simulink model "c28069pmsmfoc_cla"  (R2021b)
settings: Solver=FixedStepDiscrete  StartTime=0.0  StopTime=inf  RelTol=1e-3  EnableMultiTasking=on
PreLoadFcn:
  | c28069pmsmfoc_data;
model workspace (MAT data in the model file):
  encoderResolution = 2000
  hallOffset = '0.5'
  indexOffset = 850
  polePairs = '4'
values from neighbouring files (symbols this model uses):
  Hall_position_offset = 0.57    [c28027pmsmfoc_data.m]    (also in c28035pmsmfoc_data.m; c28035pmsmfoc_data_cla.m; c28069pmsmfoc_data.m)
  PWM_Counter_Period = CPU_frequency/PWM_frequency/2    (= 1500)    [c28027pmsmfoc_data.m]    (also in c28035pmsmfoc_data.m; c28035pmsmfoc_data_cla.m = 2500; c28069pmsmfoc_data.m = 2250)
  Speed_per_unit_scaler = 1200    [c28027pmsmfoc_data.m]    (also in c28035pmsmfoc_data.m; c28035pmsmfoc_data_cla.m = 600; c28069pmsmfoc_data.m)
  Speed_rpm_scaler = 60*CPU_frequency/Pole_pairs/2    (= 450000000)    [c28027pmsmfoc_data.m]    (also in c28035pmsmfoc_data.m; c28035pmsmfoc_data_cla.m; c28069pmsmfoc_data.m = 675000000)
undefined symbols (not defined in the file or in its folder): codertarget, Down, GPTRIP1SEL, GPTRIP2SEL, TZ1, TZ2, Up
libraries: idelinklib_common x12, c2802xlib x7, tiiqmathlib x7, hall_sensor_lib x7, c280xlib x3, c2803xlib x2, simulink x2, etargetslib x2, demo_controls x1, c2806xlib x1, c2000lib x1
(part 2 of 3)

== system c28069pmsmfoc_cla/FOC Algorithm/Torque Control Algorithm/Atomic Hall Reading ==
  Disable Interrupts for Atomic Read : Subsystem  mask(System Outputs){ShowInLibBrowser=0}
      mask prompts: ShowInLibBrowser "Simulink:masks:CustCodeMaskParam1_MP"
      settings: CopyFcn=cccopyfcn(gcb)  OpenFcn=ccopenfcn('System Outputs Function')
      mask Help: eval('feval(''rtwprivate'',''rtwhelpview'',''rtw_sys_outputs_block'')');
      mask Display: disp('System\nOutputs');
  Read Global Direction Flag : DataStoreRead  DataStoreName=Global_direction  IndexOptions=Index vector (dialog)  Indices=1  OutputSizes=1
  Read Global Speed : DataStoreRead  DataStoreName=Global_speed  IndexOptions=Index vector (dialog)  Indices=1  OutputSizes=1
  Read Global Speed and Direction Valid Flag : DataStoreRead  DataStoreName=Global_speed_and_direction_valid_flag  IndexOptions=Index vector (dialog)  Indices=1  OutputSizes=1
  Read Hall Watchdog : DataStoreRead  DataStoreName=Hall_Watchdog  IndexOptions=Index vector (dialog)  Indices=1  OutputSizes=1
  Read Halls : hall_sensor_lib/Read_halls  sample_time=-1
      settings: SourceProductBaseCode=TIC2000
  Update Hall Watchdog : Subsystem
  Direction : Outport
  Valid Flag : Outport  Port=2
  Speed : Outport  Port=3
  Halls : Outport  Port=4
  Hall Watchdog : Outport  Port=5
  wires:
  Read Hall Watchdog/1 -> Hall Watchdog/1, Update Hall Watchdog/1(In1)
  Read Halls/1 -> Halls/1
  Read Global Speed/1 -> Speed/1
  Read Global Speed and Direction Valid Flag/1 -> Valid Flag/1
  Read Global Direction Flag/1 -> Direction/1

== system c28069pmsmfoc_cla/FOC Algorithm/Torque Control Algorithm/Direction Scaling ==
  Dir : Inport
  Bias : Bias  Bias=1
  Binary Direction : Outport
  wires:
  Bias/1 -> Binary Direction/1
  Dir/1 -> Bias/1

== system c28069pmsmfoc_cla/FOC Algorithm/Torque Control Algorithm/Generating Space Vectors ==
  Speed/Pos/Dir : Inport
  Ia : Inport  Port=2
  Ib : Inport  Port=3
  Iq Desired : Inport  Port=4
  CLA Task : c2806xlib/CLA Task  taskNumber=1  intSource=Software  sampleTime=-1  claType=0  softTrigSelected=1  enableInterrupt=on
      settings: SourceProductBaseCode=TIC2000
  Data Type Conversion{1..3,7} (4 alike) : DataTypeConversion  OutDataTypeStr=single
  Generating Raw Space Vectors : Subsystem  Tag=ClaSubsystem  InitFcn=codertarget.registry.registerC28xNonPeripheralBlocks(gcb)  TreatAsAtomicUnit=on  RTWFileName=sample_cla  mask(c28x CLA Subsystem){}
      settings: CopyFcn=codertarget.registry.setC28xCLASubSystem(gcb)  OpenFcn=open_system(gcbh,'force')  RTWSystemCode=Nonreusable function  RTWFileNameOpts=User specified  FunctionWithSeparateData=on  RTWMemSecFuncInitTerm=C28xFunction  RTWMemSecFuncExecute=ClaFunction  RTWMemSecDataConstants=Cla1DataRam  RTWMemSecDataInternal=Cla1DataRam  RTWMemSecDataParameters=Cla1DataRam
      mask Display: color('black'); text(0.50, 0.12, 'CLA Subsystem', 'horizontalAlignment','center');
  Selector : Selector  InputPortWidth=3  IndexOptions=Index vector (dialog)  Indices=2  OutputSizes=1
  wires:
  Ib/1 -> Data Type Conversion1/1
  Data Type Conversion2/1 -> Generating Raw Space Vectors/1(Ia)
  Iq Desired/1 -> Data Type Conversion7/1
  CLA Task/1 -> Generating Raw Space Vectors/Trigger
  Data Type Conversion1/1 -> Generating Raw Space Vectors/2(Ib)
  Data Type Conversion3/1 -> Generating Raw Space Vectors/3(position)
  Data Type Conversion7/1 -> Generating Raw Space Vectors/4(iQ_desired)
  Selector/1 -> Data Type Conversion3/1
  Ia/1 -> Data Type Conversion2/1
  Speed/Pos/Dir/1 -> Selector/1

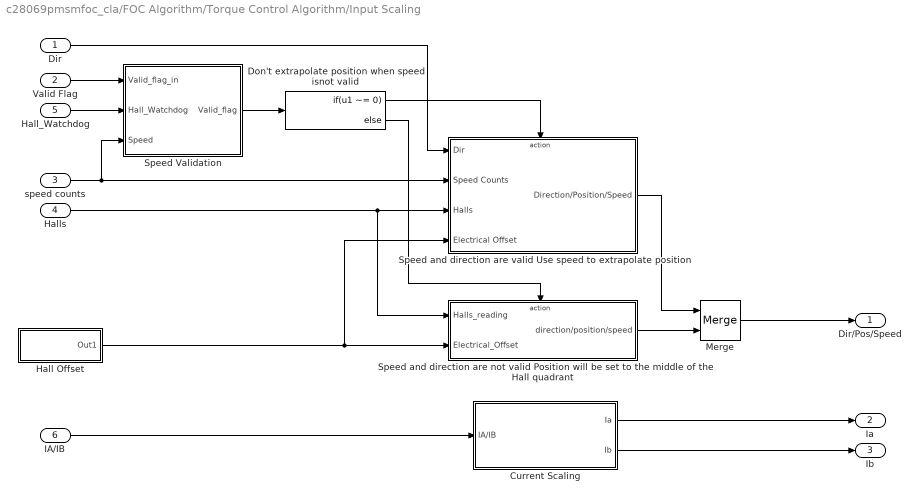
== system c28069pmsmfoc_cla/FOC Algorithm/Torque Control Algorithm/Input Scaling ==
  Dir : Inport
  Valid Flag : Inport  Port=2
  speed counts : Inport  Port=3
  Halls : Inport  Port=4
  Hall_Watchdog : Inport  Port=5
  IA/IB : Inport  Port=6
  Current Scaling : Subsystem
  Don't extrapolate position when speed isnot valid : If  IfExpression=u1 ~= 0
  Hall Offset : Subsystem
  Merge : Merge
  Speed Validation : Subsystem
  Speed and direction are not valid Position will be set to the middle of the Hall quadrant : Subsystem  TreatAsAtomicUnit=on
  Speed and direction are valid Use speed to extrapolate position : Subsystem  TreatAsAtomicUnit=on
  Dir/Pos/Speed : Outport  InitialOutput=0
  Ia : Outport  Port=2
  Ib : Outport  Port=3
  wires:
  IA/IB/1 -> Current Scaling/1(IA/IB)
  Current Scaling/2(Ib) -> Ib/1
  Current Scaling/1(Ia) -> Ia/1
  Hall_Watchdog/1 -> Speed Validation/2(Hall_Watchdog)
  Speed and direction are not valid Position will be set to the middle of the Hall quadrant/1(direction/position/speed) -> Merge/2
  Speed and direction are valid Use speed to extrapolate position/1(Direction/Position/Speed) -> Merge/1
  Speed Validation/1(Valid_flag) -> Don't extrapolate position when speed isnot valid/1
  Merge/1 -> Dir/Pos/Speed/1
  Don't extrapolate position when speed isnot valid/1 -> Speed and direction are valid Use speed to extrapolate position/Action
  Valid Flag/1 -> Speed Validation/1(Valid_flag_in)
  Halls/1 -> Speed and direction are valid Use speed to extrapolate position/3(Halls), Speed and direction are not valid Position will be set to the middle of the Hall quadrant/1(Halls_reading)
  speed counts/1 -> Speed Validation/3(Speed), Speed and direction are valid Use speed to extrapolate position/2(Speed Counts)
  Dir/1 -> Speed and direction are valid Use speed to extrapolate position/1(Dir)
  Hall Offset/1(Out1) -> Speed and direction are not valid Position will be set to the middle of the Hall quadrant/2(Electrical_Offset), Speed and direction are valid Use speed to extrapolate position/4(Electrical Offset)
  Don't extrapolate position when speed isnot valid/2 -> Speed and direction are not valid Position will be set to the middle of the Hall quadrant/Action

== system c28069pmsmfoc_cla/FOC Algorithm/Torque Control Algorithm/Send to DAC 3 ==
  Position : Inport
  Bitwise Operator : simulink/Logic and Bit Operations/Bitwise Operator  logicop=AND  UseBitMask=on  BitMask=hex2dec('0FFF')  BitMaskRealWorld=Stored Integer
  DAC 3 : c2802xlib/ePWM  PwmType=C2000  useModule=ePWM5  ePWMxLINKTBPRD=Not Linked  periodUnits=Clock cycles  timerSource=Specify via dialog  timerPeriod_clk=4095  timerPeriod_sec=64000  tbshadow=Counter equals to zero  countingMode=Up  phaseActiveEnable=Disable  phaseDirection=Count down after sync  phaseActive=0  synchronizationEnable=off  dcaevt1Sync=off  dcbevt1Sync=off  synchronizationOption=Disable  perSynchronizationOption=Counter equals to period (CTR=PRD)  clockPrescale=1  HSclockPrescale=1  enswap=off  ePWMxAStatus=on  ePWMxAactionLogic1=Do nothing  ePWMxAactionLogic2=Set  ePWMxAactionLogic3=Clear  ePWMxAactionLogic4=Do nothing  ePWMxAactionLogic5=Do nothing  ePWMxAactionLogic6=Do nothing  ePWMxACSFenable=off  ePWMxACSFvalue=Forcing disable  ePWMxASFreload=Zero  ePWMxBStatus=off  ePWMxBactionLogic1=Do nothing  ePWMxBactionLogic2=Set  ePWMxBactionLogic3=Do nothing  ePWMxBactionLogic4=Do nothing  ePWMxBactionLogic5=Clear  ePWMxBactionLogic6=Do nothing  ePWMxBCSFenable=off  ePWMxBCSFvalue=Forcing disable  ePWMxBSFreload=Zero  ePWNxBOutWay=off  ePWMxLINKCMPA=Not Linked  CMPAUnits=Clock cycles  CMPASource=Input port  CMPAValue_per=32000  CMPAValue_clk=0  enCMPAshadow=Counter equals to zero (CTR=Zero)  ePWMxLINKCMPB=Not Linked  CMPBUnits=Clock cycles  CMPBSource=Specify via dialog  CMPBValue_per=50  CMPBValue_clk=0  enCMPBshadow=Counter equals to zero (CTR=Zero)  ePWMxLINKCMPC=Not Linked  CMPCUnits=Clock cycles  CMPCSource=Specify via dialog  CMPCValue_per=50  CMPCValue_clk=32000  enCMPCshadow=Counter equals to zero (CTR=Zero)  ePWMxLINKCMPD=Not Linked  CMPDUnits=Clock cycles  CMPDSource=Specify via dialog  CMPDValue_per=50  CMPDValue_clk=32000  enCMPDshadow=Counter equals to zero (CTR=Zero)  enableDBePWMxA=off  enableDBePWMxB=off  enhalfcycle=off  DBpolarity=Active high (AH)  DBedgeDelay=Positive  DBSource_ePWMxA=ePWMxA  DBSource_ePWMxB=ePWMxA  DBPeriodUnits=Clock cycles  DBperiodSource=Specify via dialog  REDperiod=0  FEDperiod=0  REDperiod_sec=0  FEDperiod_sec=0  LoadModeDBRED=Immediate without using shadow  LoadModeDBFED=Immediate without using shadow  adcstartModuleA=off  adcrequestEventA=First event  adcstartEventA=Digital Compare Module A Event 1 start of conversion (DCAEVT1.soc)  adcstartEventA_type2=Digital Compare Module A Event 1 start of conversion (DCAEVT1.soc)  adcstartModuleB=off  adcrequestEventB=First event  adcstartEventB=Counter equals to zero (CTR=Zero)  adcstartEventB_type2=Counter equals to zero (CTR=Zero)  intEn=off  intPrd=First event  intSel=Counter equals to zero (CTR=Zero)  intSel_type2=Counter equals to zero (CTR=Zero)  hrpe=off  enHRPWM=off  HRPWM_LoadMode=Counter equals to period (CTR=PRD)  HRPWM_CTLMode=Duty or Period control mode  HRPWM_EDGMode=Both edge  hrpeb=off  enHRPWMB=off  HRPWM_LoadModeB=Counter equals to zero (CTR=ZERO)  HRPWM_CTLModeB=Duty or Period control mode  HRPWM_EDGModeB=Both edge  enHRDBRED=off  enHRDBFED=off  enSFO=on  enautoconv=on  chopperEnable=off  chopperFrequency=1  chopperFirstwidth=1  chopperDuty=12.5%  tripZonesource=Specify via dialog  tzselOSHT1=off  tzselOSHT2=off  tzselOSHT3=off  tzselOSHDCAEV1=off  tzselOSHDCBEV1=off  tzselCBC1=off  tzselCBC2=off  tzselCBC3=off  tzselCBCDCAEV2=off  tzselCBCDCBEV2=off  tzselOSHT4=off  tzselOSHT5=off  tzselOSHT6=off  tzselCBC4=off  tzselCBC5=off  tzselCBC6=off  enTzOstIntr=off  enTzCbcIntr=off  enTzDCAEVT1Intr=off  enTzDCAEVT2Intr=off  enTzDCBEVT1Intr=off  enTzDCBEVT2Intr=off  ePWMxAforced=No action  ePWMxBforced=No action  DCAEVT1forced=No action  DCBEVT1forced=No action  DCAEVT2forced=No action  DCBEVT2forced=No action  dcah=Trip Zone 1 input (TZ1)  dcal=Trip Zone 2 input (TZ2)  dcbh=Trip Zone 1 input (TZ1)  dcbl=Trip Zone 2 input (TZ2)  dcah_type2=GPTRIP1SEL/(TZ1)  dcal_type2=GPTRIP2SEL/(TZ2)  dcbh_type2=GPTRIP1SEL/(TZ1)  dcbl_type2=GPTRIP2SEL/(TZ2)  gendcaevt1=Event disabled  gendcaevt2=Event disabled  gendcbevt1=Event disabled  gendcbevt2=Event disabled  dcaevt1src=DCAEVT1 with sync  dcaevt2src=DCAEVT2 with sync  dcbevt1src=DCBEVT1 with sync  dcbevt2src=DCBEVT2 with sync  pulsesel=Counter equals to zero (CTR=Zero)  blankinv=off  blankoffset=0  blankwidth=0  evsrcsel=Filtered version of DCAEVT1 (DCAEVT1FILT)  encape=off
  Data Type Conversion : DataTypeConversion  OutDataTypeStr=uint16  ConvertRealWorld=Stored Integer (SI)
  Shift Arithmetic2 : ArithShift  BitShiftNumber=5  BitShiftDirection=Right
  wires:
  Shift Arithmetic2/1 -> Data Type Conversion/1
  Data Type Conversion/1 -> Bitwise Operator/1
  Position/1 -> Shift Arithmetic2/1
  Bitwise Operator/1 -> DAC 3/1

== system c28069pmsmfoc_cla/FOC Algorithm/Torque Control Algorithm/Speed IIR filter ==
  Speed : Inport
  Add : Sum  Inputs=+-
  Add1 : Sum
  Constant1 : Constant  OutDataTypeStr=fixdt(1,32,17)
  Constant2 : Constant  Value=.01  OutDataTypeStr=fixdt(1,32,17)
  Product : Product  OutDataTypeStr=Inherit: Same as first input
  Product1 : Product  OutDataTypeStr=Inherit: Same as first input
  Unit Delay : UnitDelay  SampleTime=-1  HasFrameUpgradeWarning=on
  Filtered speed : Outport
  wires:
  Speed/1 -> Product/1
  Add1/1 -> Unit Delay/1, Filtered speed/1
  Constant1/1 -> Add/1
  Constant2/1 -> Product/2, Add/2
  Product/1 -> Add1/1
  Add/1 -> Product1/1
  Unit Delay/1 -> Product1/2
  Product1/1 -> Add1/2

== system c28069pmsmfoc_cla/Hall Sensor A/Overflow Detection/No overflow detected ==
  old_validate : Inport
  Action Port : ActionPort  ActionPortLabel=else
  Unit Delay3 : UnitDelay  SampleTime=-1  HasFrameUpgradeWarning=on
  New_valid_flag : Outport
  wires:
  old_validate/1 -> Unit Delay3/1
  Unit Delay3/1 -> New_valid_flag/1

== system c28069pmsmfoc_cla/Hall Sensor A/Overflow Detection/Overflow detected ==
  Action Port : ActionPort  ActionPortLabel=if(u1 ~= 0)
  Constant : Constant  Value=0  OutDataTypeStr=uint16
  Constant2 : Constant  Value=0  OutDataTypeStr=uint16
  Data Store : DataStoreWrite  DataStoreName=Global_speed_and_direction_valid_flag  IndexOptions=Index vector (dialog)  Indices=1  OutputSizes=1
  New_valid_flag : Outport
  wires:
  Constant/1 -> New_valid_flag/1
  Constant2/1 -> Data Store/1

== system c28069pmsmfoc_cla/Hall Sensor A/Update Speed and Direction/update_speed ==
  In1 : Inport
  Action Port : ActionPort  ActionPortLabel=if(u1 ~= 0)
  Data Store Write3 : DataStoreWrite  DataStoreName=Global_speed  IndexOptions=Index vector (dialog)  Indices=1  OutputSizes=1
  wires:
  In1/1 -> Data Store Write3/1

== system c28069pmsmfoc_cla/Hall Sensor B/Overflow Detection/No overflow detected ==
  old_validate : Inport
  Action Port : ActionPort  ActionPortLabel=else
  Unit Delay3 : UnitDelay  SampleTime=-1  HasFrameUpgradeWarning=on
  New_valid_flag : Outport
  wires:
  Unit Delay3/1 -> New_valid_flag/1
  old_validate/1 -> Unit Delay3/1

== system c28069pmsmfoc_cla/Hall Sensor B/Overflow Detection/Overflow detected ==
  Action Port : ActionPort  ActionPortLabel=if(u1 ~= 0)
  Constant : Constant  Value=0  OutDataTypeStr=uint16
  Constant2 : Constant  Value=0  OutDataTypeStr=uint16
  Data Store : DataStoreWrite  DataStoreName=Global_speed_and_direction_valid_flag  IndexOptions=Index vector (dialog)  Indices=1  OutputSizes=1
  New_valid_flag : Outport
  wires:
  Constant2/1 -> Data Store/1
  Constant/1 -> New_valid_flag/1

== system c28069pmsmfoc_cla/Hall Sensor B/Update Speed and Direction/update_speed ==
  In1 : Inport
  Action Port : ActionPort  ActionPortLabel=if(u1 ~= 0)
  Data Store Write3 : DataStoreWrite  DataStoreName=Global_speed  IndexOptions=Index vector (dialog)  Indices=1  OutputSizes=1
  wires:
  In1/1 -> Data Store Write3/1

== system c28069pmsmfoc_cla/Hall Sensor C/Overflow Detection/No overflow detected ==
  old_validate : Inport
  Action Port : ActionPort  ActionPortLabel=else
  Unit Delay3 : UnitDelay  SampleTime=-1  HasFrameUpgradeWarning=on
  New_valid_flag : Outport
  wires:
  old_validate/1 -> Unit Delay3/1
  Unit Delay3/1 -> New_valid_flag/1

== system c28069pmsmfoc_cla/Hall Sensor C/Overflow Detection/Overflow detected ==
  Action Port : ActionPort  ActionPortLabel=if(u1 ~= 0)
  Constant : Constant  Value=0  OutDataTypeStr=uint16
  Constant2 : Constant  Value=0  OutDataTypeStr=uint16
  Data Store : DataStoreWrite  DataStoreName=Global_speed_and_direction_valid_flag  IndexOptions=Index vector (dialog)  Indices=1  OutputSizes=1
  New_valid_flag : Outport
  wires:
  Constant/1 -> New_valid_flag/1
  Constant2/1 -> Data Store/1

== system c28069pmsmfoc_cla/Hall Sensor C/Update Speed and Direction/update_speed ==
  In1 : Inport
  Action Port : ActionPort  ActionPortLabel=if(u1 ~= 0)
  Data Store Write3 : DataStoreWrite  DataStoreName=Global_speed  IndexOptions=Index vector (dialog)  Indices=1  OutputSizes=1
  wires:
  In1/1 -> Data Store Write3/1

== system c28069pmsmfoc_cla/Speed Controller/PID Controller/UD_REG3 ==
  up_reg3 : Inport
  PrevOut : Inport  Port=2
  Constant : Constant  Value=derivativeGain  OutDataTypeStr=Inherit: Inherit via back propagation
  Product : Product  OutDataTypeStr=Inherit: Same as first input
  Sum2 : Sum  Inputs=+-
  Out1 : Outport
  wires:
  Constant/1 -> Product/1
  Product/1 -> Out1/1
  Sum2/1 -> Product/2
  PrevOut/1 -> Sum2/2
  up_reg3/1 -> Sum2/1

== system c28069pmsmfoc_cla/Speed Controller/PID Controller/UI_REG3 ==
  OLD_UI_REG3 : Inport
  up_reg3 : Inport  Port=2
  saterr_reg3 : Inport  Port=3
  Constant : Constant  Value=integralGain  OutDataTypeStr=Inherit: Inherit via back propagation
  Constant1 : Constant  Value=correctionGain  OutDataTypeStr=Inherit: Inherit via back propagation
  Product : Product  OutDataTypeStr=Inherit: Same as first input
  Product1 : Product  OutDataTypeStr=Inherit: Same as first input
  Sum1 : Sum  Inputs=+++
  UI_REG1 : Outport
  wires:
  Constant1/1 -> Product1/1
  saterr_reg3/1 -> Product1/2
  Constant/1 -> Product/1
  up_reg3/1 -> Product/2
  Sum1/1 -> UI_REG1/1
  Product1/1 -> Sum1/3
  Product/1 -> Sum1/2
  OLD_UI_REG3/1 -> Sum1/1

== system c28069pmsmfoc_cla/FOC Algorithm/Torque Control Algorithm/Atomic Hall Reading/Disable Interrupts for Atomic Read ==

== system c28069pmsmfoc_cla/FOC Algorithm/Torque Control Algorithm/Atomic Hall Reading/Update Hall Watchdog ==
  In1 : Inport
  Add : Sum  SaturateOnIntegerOverflow=on
      settings: AttributesFormatString=Saturation: %<SaturateOnIntegerOverflow>
  Constant2 : Constant  OutDataTypeStr=uint16
  Write Hall Watchdog : DataStoreWrite  DataStoreName=Hall_Watchdog  IndexOptions=Index vector (dialog)  Indices=1  OutputSizes=1
  wires:
  Add/1 -> Write Hall Watchdog/1
  Constant2/1 -> Add/2
  In1/1 -> Add/1

== system c28069pmsmfoc_cla/FOC Algorithm/Torque Control Algorithm/Generating Space Vectors/Generating Raw Space Vectors ==
  Ia : Inport
  Ib : Inport  Port=2
  position : Inport  Port=3
  iQ_desired : Inport  Port=4
  function : TriggerPort  TriggerType=function-call  VariantControl=Variant
  Clarke Transformation : Subsystem  InitFcn=tic2000lib_licenseCheck  mask(Clarke Transformation){}
      mask help: This block performs transformation of three-phase quantities into balanced two-phase quadrature quantities. All inputs and outputs are signed 32-bit fixed-point numbers with Q value between 1 and 29.
      mask Help: eval('linkfoundation.util.openBlockHelp(''c28xdmclibclarketransformation'',''ecoder'')');
      mask Display:
      | port_label('input',1,'As');
      | port_label('input',2,'Bs');
      | port_label('Output',1,'Alpha');
      | port_label('Output',2,'Beta');
      | text(0.5,0.15, 'Clarke', 'horizontalalignment','center');
  Data Store Write : DataStoreWrite  DataStoreName=Ta_out  IndexOptions=Index vector (dialog)  Indices=1  OutputSizes=1
  Data Store Write1 : DataStoreWrite  DataStoreName=Tb_out  IndexOptions=Index vector (dialog)  Indices=1  OutputSizes=1
  Data Store Write2 : DataStoreWrite  DataStoreName=Tc_out  IndexOptions=Index vector (dialog)  Indices=1  OutputSizes=1
  Inverse Park Transformation : Subsystem  InitFcn=tic2000lib_licenseCheck  mask(Inverse Park Transformation){}
      mask help: This block performs vector transformation from orthogonal rotating reference frame into orthogonal stationary frame. All inputs and outputs are signed 32-bit fixed-point numbers with Q value between 1 and 29.
      mask Help: eval('linkfoundation.util.openBlockHelp(''c28xdmclibinverseparktransformation'',''ecoder'')');
      mask Display:
      | port_label('input',1,'Ds');
      | port_label('input',2,'Qs');
      | port_label('input',3,'Angle');
      | port_label('Output',1,'Alpha');
      | port_label('Output',2,'Beta');
      | text(0.5,0.15, 'IPark', 'horizontalalignment','center');
  Park Transformation : Subsystem  InitFcn=tic2000lib_licenseCheck  mask(Park Transformation){}
      mask help: This block performs vector transformation from balanced two-phase orthogonal stationary system into orthogonal rotating frame. All inputs and outputs are signed 32-bit fixed-point numbers with Q value between 1 and 29.
      mask Help: eval('linkfoundation.util.openBlockHelp(''c28xdmclibparktransformation'',''ecoder'')');
      mask Display:
      | port_label('input',1,'Alpha');
      | port_label('input',2,'Beta');
      | port_label('input',3,'Angle');
      | port_label('Output',1,'Ds');
      | port_label('Output',2,'Qs');
      | text(0.5,0.15, 'Park', 'horizontalalignment','center');
  SVGen : Subsystem
  control : Subsystem
  wires:
  control/1(Out1) -> Inverse Park Transformation/1(ID)
  iQ_desired/1 -> control/3(Iq desired)  "iQ_des"
  Ib/1 -> Clarke Transformation/2(Ib)  "Ib_in"
  Ia/1 -> Clarke Transformation/1(Ia)  "Ia_in"
  control/2(Out2) -> Inverse Park Transformation/2(IQ)
  Inverse Park Transformation/1(Out1) -> SVGen/1(Ua)
  Clarke Transformation/2(Out2) -> Park Transformation/2(Iq1)
  Clarke Transformation/1(Out1) -> Park Transformation/1(Id1)
  SVGen/3(Tc) -> Data Store Write2/1
  SVGen/1(Ta) -> Data Store Write/1
  position/1 -> Inverse Park Transformation/3(theta), Park Transformation/3(theta1)  "position"
  Inverse Park Transformation/2(Out2) -> SVGen/2(Ub)
  Park Transformation/2(Out4) -> control/2(Vq)
  SVGen/2(Tb) -> Data Store Write1/1
  Park Transformation/1(Out3) -> control/1(Vd)

== system c28069pmsmfoc_cla/FOC Algorithm/Torque Control Algorithm/Input Scaling/Current Scaling ==
  IA/IB : Inport
  Add : Sum  Inputs=-+
  Constant : Constant  Value=[2048 2048]  OutDataTypeStr=int32
  Data Type Conversion : DataTypeConversion  OutDataTypeStr=int32  ConvertRealWorld=Stored Integer (SI)
  Data Type Conversion1 : DataTypeConversion  OutDataTypeStr=fixdt(1,32,17)  ConvertRealWorld=Stored Integer (SI)
  Demux : Demux  Outputs=2
  Shift Arithmetic : ArithShift  BitShiftNumber=-6
  Ia : Outport
  Ib : Outport  Port=2
  wires:
  IA/IB/1 -> Data Type Conversion/1
  Constant/1 -> Add/1
  Data Type Conversion1/1 -> Demux/1
  Shift Arithmetic/1 -> Data Type Conversion1/1
  Add/1 -> Shift Arithmetic/1
  Data Type Conversion/1 -> Add/2
  Demux/2 -> Ib/1
  Demux/1 -> Ia/1

== system c28069pmsmfoc_cla/FOC Algorithm/Torque Control Algorithm/Input Scaling/Hall Offset ==
  Hall_offset : Constant  Value=Hall_position_offset  OutDataTypeStr=fixdt(1,32,17)
  Out1 : Outport
  wires:
  Hall_offset/1 -> Out1/1

== system c28069pmsmfoc_cla/FOC Algorithm/Torque Control Algorithm/Input Scaling/Speed Validation ==
  Valid_flag_in : Inport
  Hall_Watchdog : Inport  Port=2
  Speed : Inport  Port=3
  Constant : Constant  Value=0  OutDataTypeStr=uint16
  Don't trust speed if Hall Watchdog counter is too high. Hall Watchdog is reset at every Hall edge. : Switch  Threshold=65000
  Don't trust speed if it is below 10rpm : Switch  Threshold=Speed_rpm_scaler/10
  Valid_flag : Outport
  wires:
  Don't trust speed if it is below 10rpm/1 -> Don't trust speed if Hall Watchdog counter is too high. Hall Watchdog is reset at every Hall edge./3
  Valid_flag_in/1 -> Don't trust speed if it is below 10rpm/3
  Speed/1 -> Don't trust speed if it is below 10rpm/2
  Don't trust speed if Hall Watchdog counter is too high. Hall Watchdog is reset at every Hall edge./1 -> Valid_flag/1
  Constant/1 -> Don't trust speed if it is below 10rpm/1, Don't trust speed if Hall Watchdog counter is too high. Hall Watchdog is reset at every Hall edge./1
  Hall_Watchdog/1 -> Don't trust speed if Hall Watchdog counter is too high. Hall Watchdog is reset at every Hall edge./2

== system c28069pmsmfoc_cla/FOC Algorithm/Torque Control Algorithm/Input Scaling/Speed and direction are not valid Position will be set to the middle of the Hall quadrant ==
  Halls_reading : Inport
  Electrical_Offset : Inport  Port=2
  Action Port : ActionPort  ActionPortLabel=else
  Add : Sum
  Direction : Constant  Value=0  OutDataTypeStr=fixdt(1,32,17)
  Extract position from Halls reading. No speed extrapolaiton : Subsystem
  Mux1 : Mux  Inputs=3
  Speed : Constant  Value=0  OutDataTypeStr=fixdt(1,32,17)
  direction/position/speed : Outport  InitialOutput=0
  wires:
  Speed/1 -> Mux1/3
  Electrical_Offset/1 -> Add/2
  Add/1 -> Mux1/2
  Extract position from Halls reading. No speed extrapolaiton/1(Raw position) -> Add/1
  Mux1/1 -> direction/position/speed/1
  Direction/1 -> Mux1/1
  Halls_reading/1 -> Extract position from Halls reading. No speed extrapolaiton/1(Halls_reading)

== system c28069pmsmfoc_cla/FOC Algorithm/Torque Control Algorithm/Input Scaling/Speed and direction are valid Use speed to extrapolate position ==
  Dir : Inport
  Speed Counts : Inport  Port=2
  Halls : Inport  Port=3
  Electrical Offset : Inport  Port=4
  Action Port : ActionPort  ActionPortLabel=if(u1 ~= 0)
  Data Type Conversion1 : DataTypeConversion  OutDataTypeStr=fixdt(1,32,17)  ConvertRealWorld=Stored Integer (SI)
  Data Type Conversion2 : DataTypeConversion  OutDataTypeStr=fixdt(1,32,17)
  Demux : Demux  Outputs=2
  Extract Position from Halls : Subsystem
  Extrapolate position : Subsystem
  Mux2 : Mux  Inputs=3
  Per unit speed calcualtion : Subsystem
  Direction/Position/Speed : Outport  InitialOutput=0
  wires:
  Mux2/1 -> Direction/Position/Speed/1
  Data Type Conversion2/1 -> Mux2/1
  Demux/2 -> Extrapolate position/3(offset)
  Demux/1 -> Extrapolate position/2(Counter)
  Extrapolate position/1(Position) -> Mux2/2
  Dir/1 -> Data Type Conversion2/1, Per unit speed calcualtion/1(Dir), Extract Position from Halls/1(Direction)
  Electrical Offset/1 -> Extrapolate position/4(electrical offset)
  Per unit speed calcualtion/1(Per Unit Speed) -> Mux2/3
  Data Type Conversion1/1 -> Extrapolate position/1(Speed Counts), Per unit speed calcualtion/2(Speed counts)
  Halls/1 -> Extract Position from Halls/2(Halls)
  Extract Position from Halls/1(Counter/Offset) -> Demux/1
  Speed Counts/1 -> Data Type Conversion1/1

== system c28069pmsmfoc_cla/FOC Algorithm/Torque Control Algorithm/Generating Space Vectors/Generating Raw Space Vectors/Clarke Transformation ==
  Ia : Inport
  Ib : Inport  Port=2
  1 : Constant  Value=0.57735026918963  OutDataTypeStr=Inherit: Inherit via back propagation
  2 : Constant  Value=2  OutDataTypeStr=Inherit: Inherit via back propagation  SampleTime=Inf
  Product : Product  OutDataTypeStr=single
  Product1 : Product  OutDataTypeStr=Inherit: Same as first input
  Sum1 : Sum  Inputs=|++  OutDataTypeStr=Inherit: Same as first input
  Out1 : Outport
  Out2 : Outport  Port=2
  wires:
  Ib/1 -> Product/2
  Ia/1 -> Out1/1, Sum1/1
  Sum1/1 -> Product1/2
  2/1 -> Product/1
  Product1/1 -> Out2/1
  Product/1 -> Sum1/2
  1/1 -> Product1/1

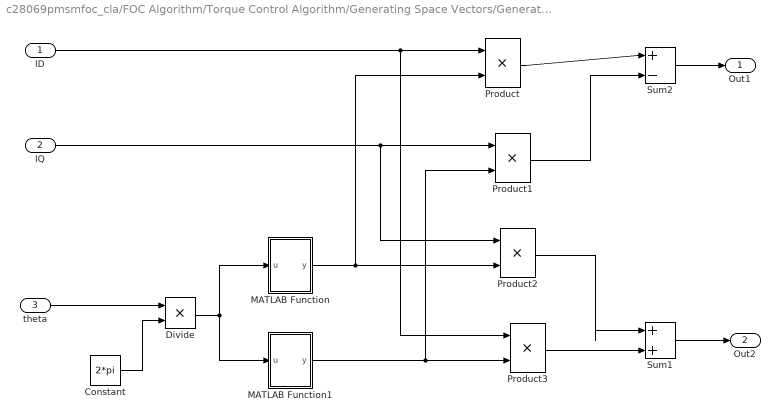
== system c28069pmsmfoc_cla/FOC Algorithm/Torque Control Algorithm/Generating Space Vectors/Generating Raw Space Vectors/Inverse Park Transformation ==
  ID : Inport
  IQ : Inport  Port=2
  theta : Inport  Port=3
  Constant : Constant  Value=2*pi  OutDataTypeStr=single
  Divide : Product  Inputs=**
  MATLAB Function : MATLAB Function  TreatAsAtomicUnit=on
  MATLAB Function1 : MATLAB Function  TreatAsAtomicUnit=on
  Product{,1..3} (4 alike) : Product  OutDataTypeStr=Inherit: Same as first input
  Sum1 : Sum  Inputs=|++  OutDataTypeStr=Inherit: Same as first input
  Sum2 : Sum  Inputs=|+-  OutDataTypeStr=Inherit: Same as first input
  Out1 : Outport
  Out2 : Outport  Port=2
  wires:
  IQ/1 -> Product2/1, Product1/1
  ID/1 -> Product3/1, Product/1
  Sum2/1 -> Out1/1
  Sum1/1 -> Out2/1
  Product1/1 -> Sum2/2
  Product2/1 -> Sum1/1
  Product/1 -> Sum2/1
  Product3/1 -> Sum1/2
  MATLAB Function1/1(y) -> Product3/2, Product1/2
  MATLAB Function/1(y) -> Product2/2, Product/2
  theta/1 -> Divide/1
  Constant/1 -> Divide/2
  Divide/1 -> MATLAB Function/1(u), MATLAB Function1/1(u)

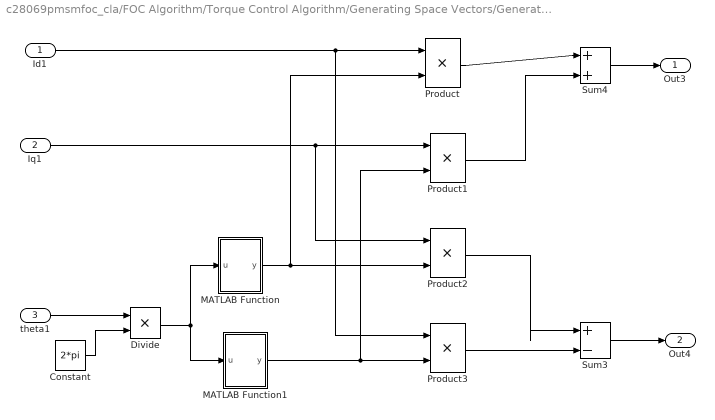
== system c28069pmsmfoc_cla/FOC Algorithm/Torque Control Algorithm/Generating Space Vectors/Generating Raw Space Vectors/Park Transformation ==
  Id1 : Inport
  Iq1 : Inport  Port=2
  theta1 : Inport  Port=3
  Constant : Constant  Value=2*pi  OutDataTypeStr=single
  Divide : Product  Inputs=**
  MATLAB Function : MATLAB Function
  MATLAB Function1 : MATLAB Function
  Product{,1..3} (4 alike) : Product  OutDataTypeStr=Inherit: Same as first input
  Sum3 : Sum  Inputs=|+-  OutDataTypeStr=Inherit: Same as first input
  Sum4 : Sum  Inputs=|++  OutDataTypeStr=Inherit: Same as first input
  Out3 : Outport
  Out4 : Outport  Port=2
  wires:
  Iq1/1 -> Product2/1, Product1/1
  Id1/1 -> Product3/1, Product/1
  MATLAB Function/1(y) -> Product2/2, Product/2
  MATLAB Function1/1(y) -> Product3/2, Product1/2
  Product3/1 -> Sum3/2
  Product/1 -> Sum4/1
  Product2/1 -> Sum3/1
  Product1/1 -> Sum4/2
  Sum3/1 -> Out4/1
  Sum4/1 -> Out3/1
  theta1/1 -> Divide/1
  Constant/1 -> Divide/2
  Divide/1 -> MATLAB Function1/1(u), MATLAB Function/1(u)

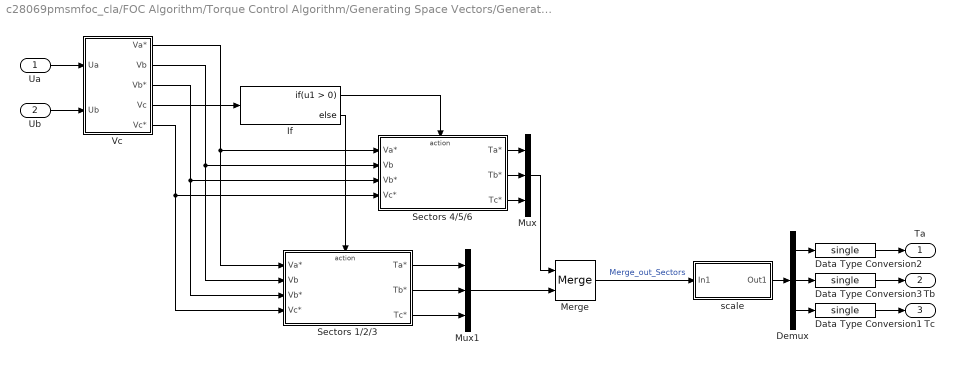
== system c28069pmsmfoc_cla/FOC Algorithm/Torque Control Algorithm/Generating Space Vectors/Generating Raw Space Vectors/SVGen ==
  Ua : Inport
  Ub : Inport  Port=2
  Data Type Conversion1 : DataTypeConversion  OutDataTypeStr=single
  Data Type Conversion2 : DataTypeConversion  OutDataTypeStr=single
  Data Type Conversion3 : DataTypeConversion  OutDataTypeStr=single
  Demux : Demux  Outputs=3
  If : If
  Merge : Merge
  Mux : Mux  Inputs=3
  Mux1 : Mux  Inputs=3
  Sectors 1/2/3 : Subsystem  TreatAsAtomicUnit=on
  Sectors 4/5/6 : Subsystem  TreatAsAtomicUnit=on
  Vc : Subsystem
  scale : Subsystem
  Ta : Outport
  Tb : Outport  Port=2
  Tc : Outport  Port=3
  wires:
  Vc/4(Vc) -> If/1
  scale/1(Out1) -> Demux/1
  Merge/1 -> scale/1(In1)  "Merge_out_Sectors"
  Sectors 4/5/6/3(Tc*) -> Mux/3
  Sectors 4/5/6/2(Tb*) -> Mux/2
  Sectors 4/5/6/1(Ta*) -> Mux/1
  Sectors 1/2/3/3(Tc*) -> Mux1/3
  Sectors 1/2/3/2(Tb*) -> Mux1/2
  Sectors 1/2/3/1(Ta*) -> Mux1/1
  Demux/3 -> Data Type Conversion1/1
  Demux/2 -> Data Type Conversion3/1
  Demux/1 -> Data Type Conversion2/1
  Mux1/1 -> Merge/2
  Mux/1 -> Merge/1
  Vc/5(Vc*) -> Sectors 1/2/3/4(Vc*), Sectors 4/5/6/4(Vc*)
  Vc/3(Vb*) -> Sectors 1/2/3/3(Vb*), Sectors 4/5/6/3(Vb*)
  Vc/2(Vb) -> Sectors 1/2/3/2(Vb), Sectors 4/5/6/2(Vb)
  Vc/1(Va*) -> Sectors 1/2/3/1(Va*), Sectors 4/5/6/1(Va*)
  If/2 -> Sectors 1/2/3/Action
  If/1 -> Sectors 4/5/6/Action
  Ua/1 -> Vc/1(Ua)
  Ub/1 -> Vc/2(Ub)
  Data Type Conversion3/1 -> Tb/1
  Data Type Conversion2/1 -> Ta/1
  Data Type Conversion1/1 -> Tc/1

== system c28069pmsmfoc_cla/FOC Algorithm/Torque Control Algorithm/Generating Space Vectors/Generating Raw Space Vectors/control ==
  Vd : Inport
  Vq : Inport  Port=2
  Iq desired : Inport  Port=3
  Constant1 : Constant  Value=0  OutDataTypeStr=single
  PID Controller : Subsystem  InitFcn=tic2000lib_licenseCheck  mask(PID Controller){proportionalGain=0.5, integralGain=0.002, correctionGain=0.002, derivativeGain=0, minOutput=-0.2, maxOutput=0.2}
      mask prompts: proportionalGain "Proportional gain:"; integralGain "Integral gain:"; correctionGain "Integral correction gain:"; derivativeGain "Derivative gain:"; minOutput "Minimum output:"; maxOutput "Maximum output:"
      mask help: This block implements a digital PID controller with anti-windup correction. Both inputs and the output are signed 32-bit fixed-point numbers with Q value between 1 and 29.
      mask init:
      | c280xDMCPIDControl_callback(proportionalGain,integralGain,correctionGain,derivativeGain,minOutput,maxOutput)
      mask Help: eval('linkfoundation.util.openBlockHelp(''c28xdmclibpidcontroller'',''ecoder'')');
      mask Display:
      | port_label('input',1,'ref');
      | port_label('input',2,'fdb');
      | port_label('Output',1,'out');
      | text(0.5,0.15, 'PID', 'horizontalalignment','center');
  PID Controller1 : Subsystem  InitFcn=tic2000lib_licenseCheck  mask(PID Controller){proportionalGain=0.5, integralGain=0.002, correctionGain=0.002, derivativeGain=0, minOutput=-0.2, maxOutput=0.2}
      mask prompts: proportionalGain "Proportional gain:"; integralGain "Integral gain:"; correctionGain "Integral correction gain:"; derivativeGain "Derivative gain:"; minOutput "Minimum output:"; maxOutput "Maximum output:"
      mask help: This block implements a digital PID controller with anti-windup correction. Both inputs and the output are signed 32-bit fixed-point numbers with Q value between 1 and 29.
      mask init:
      | c280xDMCPIDControl_callback(proportionalGain,integralGain,correctionGain,derivativeGain,minOutput,maxOutput)
      mask Help: eval('linkfoundation.util.openBlockHelp(''c28xdmclibpidcontroller'',''ecoder'')');
      mask Display:
      | port_label('input',1,'ref');
      | port_label('input',2,'fdb');
      | port_label('Output',1,'out');
      | text(0.5,0.15, 'PID', 'horizontalalignment','center');
  saturation : Subsystem
  Out1 : Outport
  Out2 : Outport  Port=2
  wires:
  Vd/1 -> PID Controller/2(In2)
  Vq/1 -> PID Controller1/2(In2)
  Iq desired/1 -> PID Controller1/1(In1)
  saturation/1(Out1) -> Out1/1
  saturation/2(Out2) -> Out2/1
  Constant1/1 -> PID Controller/1(In1)
  PID Controller/1(Out1) -> saturation/1(In1)
  PID Controller1/1(Out1) -> saturation/2(In2)

== system c28069pmsmfoc_cla/FOC Algorithm/Torque Control Algorithm/Input Scaling/Speed and direction are not valid Position will be set to the middle of the Hall quadrant/Extract position from Halls reading. No speed extrapolaiton ==
  Halls_reading : Inport
  Hall Value of 1 : Subsystem  TreatAsAtomicUnit=on
  Hall Value of 2 : Subsystem  TreatAsAtomicUnit=on
  Hall Value of 3 : Subsystem  TreatAsAtomicUnit=on
  Hall Value of 4 : Subsystem  TreatAsAtomicUnit=on
  Hall Value of 5 : Subsystem  TreatAsAtomicUnit=on
  Hall Value of 6 : Subsystem  TreatAsAtomicUnit=on
  Merge : Merge  Inputs=6
  Switch Case : SwitchCase  CaseConditions={1,2,3,4,5,6}  ShowDefaultCase=off
  Raw position : Outport
  wires:
  Hall Value of 6/1(position) -> Merge/6
  Hall Value of 5/1(position) -> Merge/5
  Hall Value of 4/1(position) -> Merge/4
  Hall Value of 3/1(position) -> Merge/3
  Hall Value of 2/1(position) -> Merge/2
  Hall Value of 1/1(position) -> Merge/1
  Switch Case/2 -> Hall Value of 2/Action
  Switch Case/5 -> Hall Value of 5/Action
  Switch Case/6 -> Hall Value of 6/Action
  Switch Case/1 -> Hall Value of 1/Action
  Switch Case/3 -> Hall Value of 3/Action
  Switch Case/4 -> Hall Value of 4/Action
  Halls_reading/1 -> Switch Case/1
  Merge/1 -> Raw position/1

== system c28069pmsmfoc_cla/FOC Algorithm/Torque Control Algorithm/Input Scaling/Speed and direction are valid Use speed to extrapolate position/Extract Position from Halls ==
  Direction : Inport
  Halls : Inport  Port=2
  Direction 0 Provides offset and counter values : Subsystem  TreatAsAtomicUnit=on
  Direction 1 Provides offset and counter values : Subsystem  TreatAsAtomicUnit=on
  Merge : Merge
  Mux : Mux  Inputs=2
  Mux1 : Mux  Inputs=2
  Switch on direction : If  IfExpression=u1 ~= 0
  Counter/Offset : Outport
  wires:
  Mux/1 -> Merge/1
  Merge/1 -> Counter/Offset/1
  Mux1/1 -> Merge/2
  Direction 0 Provides offset and counter values/2(offset) -> Mux1/2
  Direction 0 Provides offset and counter values/1(counter) -> Mux1/1
  Direction 1 Provides offset and counter values/2(offset) -> Mux/2
  Direction 1 Provides offset and counter values/1(counter) -> Mux/1
  Halls/1 -> Direction 0 Provides offset and counter values/1(halls), Direction 1 Provides offset and counter values/1(halls)
  Switch on direction/2 -> Direction 0 Provides offset and counter values/Action
  Switch on direction/1 -> Direction 1 Provides offset and counter values/Action
  Direction/1 -> Switch on direction/1

== system c28069pmsmfoc_cla/FOC Algorithm/Torque Control Algorithm/Input Scaling/Speed and direction are valid Use speed to extrapolate position/Extrapolate position ==
  Speed Counts : Inport
  Counter : Inport  Port=2
  offset : Inport  Port=3
  electrical offset : Inport  Port=4
  Add : Sum  Inputs=+++
  IQN / IQN : tiiqmathlib/IQN // IQN
      settings: SourceProductBaseCode=TIC2000
  IQN x IQN : tiiqmathlib/IQN x IQN  multiplyOption=Multiply
      settings: SourceProductBaseCode=TIC2000
  Saturate IQN1 : tiiqmathlib/Saturate IQN  pos=1/6  neg=-1/6
      settings: SourceProductBaseCode=TIC2000
  Speed is measured for half an electrical revolution : Constant  Value=1/2  OutDataTypeStr=fixdt(1,32,17)
  Position : Outport
  wires:
  electrical offset/1 -> Add/3
  Saturate IQN1/1 -> Add/1
  Speed Counts/1 -> IQN / IQN/2
  offset/1 -> Add/2
  Add/1 -> Position/1
  IQN x IQN/1 -> Saturate IQN1/1
  Speed is measured for half an electrical revolution/1 -> IQN x IQN/2
  IQN / IQN/1 -> IQN x IQN/1
  Counter/1 -> IQN / IQN/1

== system c28069pmsmfoc_cla/FOC Algorithm/Torque Control Algorithm/Input Scaling/Speed and direction are valid Use speed to extrapolate position/Per unit speed calcualtion ==
  Dir : Inport
  Speed counts : Inport  Port=2
  " IQN" : tiiqmathlib/IQN // IQN
      settings: SourceProductBaseCode=TIC2000
  Bias : Bias  Bias=1
  Constant : Constant  Value=Speed_rpm_scaler/Speed_per_unit_scaler  OutDataTypeStr=int32  LockScale=on
  Data Type Conversion1 : DataTypeConversion  OutDataTypeStr=fixdt(1,32,17)  ConvertRealWorld=Stored Integer (SI)
  Gain : Gain  Gain=-2  ParamDataTypeStr=int32  OutDataTypeStr=fixdt(1,32,17)
  mpy : Product  Inputs=**  OutDataTypeStr=fixdt(1,32,17)
  Per Unit Speed : Outport
  wires:
  Gain/1 -> Bias/1
  Constant/1 -> Data Type Conversion1/1
  " IQN"/1 -> mpy/2
  Bias/1 -> mpy/1
  Speed counts/1 -> " IQN"/2
  Data Type Conversion1/1 -> " IQN"/1
  Dir/1 -> Gain/1
  mpy/1 -> Per Unit Speed/1

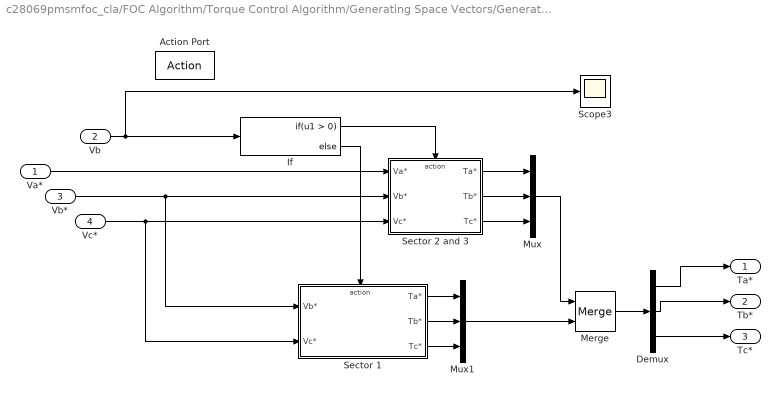
== system c28069pmsmfoc_cla/FOC Algorithm/Torque Control Algorithm/Generating Space Vectors/Generating Raw Space Vectors/SVGen/Sectors 1//2//3 ==
  Va* : Inport
  Vb : Inport  Port=2
  Vb* : Inport  Port=3
  Vc* : Inport  Port=4
  Action Port : ActionPort  ActionPortLabel=else
  Demux : Demux  Outputs=3
  If : If
  Merge : Merge
  Mux : Mux  Inputs=3
  Mux1 : Mux  Inputs=3
  Scope3 : Scope
  Sector 1 : Subsystem  TreatAsAtomicUnit=on
  Sector 2 and 3 : Subsystem  TreatAsAtomicUnit=on
  Ta* : Outport
  Tb* : Outport  Port=2
  Tc* : Outport  Port=3
  wires:
  Vb/1 -> If/1, Scope3/1
  If/1 -> Sector 2 and 3/Action
  If/2 -> Sector 1/Action
  Sector 2 and 3/1(Ta*) -> Mux/1
  Sector 2 and 3/2(Tb*) -> Mux/2
  Sector 2 and 3/3(Tc*) -> Mux/3
  Mux/1 -> Merge/1
  Mux1/1 -> Merge/2
  Merge/1 -> Demux/1
  Demux/1 -> Ta*/1
  Demux/2 -> Tb*/1
  Demux/3 -> Tc*/1
  Sector 1/1(Ta*) -> Mux1/1
  Sector 1/2(Tb*) -> Mux1/2
  Sector 1/3(Tc*) -> Mux1/3
  Va*/1 -> Sector 2 and 3/1(Va*)
  Vb*/1 -> Sector 1/1(Vb*), Sector 2 and 3/2(Vb*)
  Vc*/1 -> Sector 1/2(Vc*), Sector 2 and 3/3(Vc*)

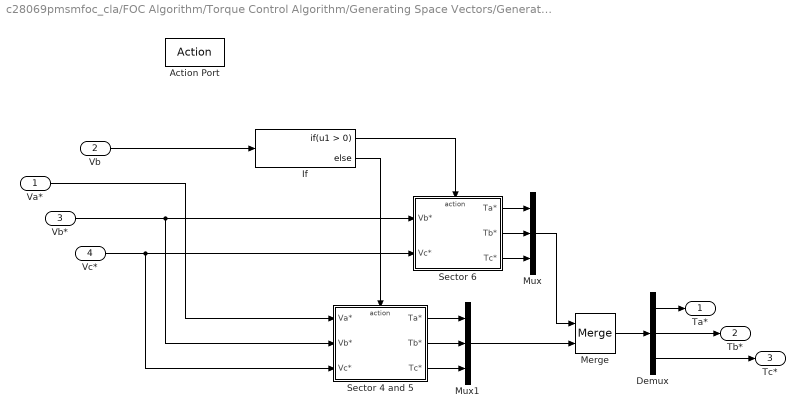
== system c28069pmsmfoc_cla/FOC Algorithm/Torque Control Algorithm/Generating Space Vectors/Generating Raw Space Vectors/SVGen/Sectors 4//5//6 ==
  Va* : Inport
  Vb : Inport  Port=2
  Vb* : Inport  Port=3
  Vc* : Inport  Port=4
  Action Port : ActionPort  ActionPortLabel=if(u1 > 0)
  Demux : Demux  Outputs=3
  If : If
  Merge : Merge
  Mux : Mux  Inputs=3
  Mux1 : Mux  Inputs=3
  Sector 4 and 5 : Subsystem  TreatAsAtomicUnit=on
  Sector 6 : Subsystem  TreatAsAtomicUnit=on
  Ta* : Outport
  Tb* : Outport  Port=2
  Tc* : Outport  Port=3
  wires:
  Vb/1 -> If/1
  Vc*/1 -> Sector 4 and 5/3(Vc*), Sector 6/2(Vc*)
  Vb*/1 -> Sector 4 and 5/2(Vb*), Sector 6/1(Vb*)
  Va*/1 -> Sector 4 and 5/1(Va*)
  Sector 4 and 5/3(Tc*) -> Mux1/3
  Sector 4 and 5/2(Tb*) -> Mux1/2
  Sector 4 and 5/1(Ta*) -> Mux1/1
  Demux/3 -> Tc*/1
  Demux/2 -> Tb*/1
  Demux/1 -> Ta*/1
  Merge/1 -> Demux/1
  Mux1/1 -> Merge/2
  Mux/1 -> Merge/1
  Sector 6/3(Tc*) -> Mux/3
  Sector 6/2(Tb*) -> Mux/2
  Sector 6/1(Ta*) -> Mux/1
  If/2 -> Sector 4 and 5/Action
  If/1 -> Sector 6/Action

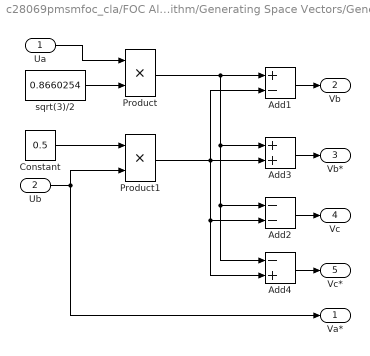
== system c28069pmsmfoc_cla/FOC Algorithm/Torque Control Algorithm/Generating Space Vectors/Generating Raw Space Vectors/SVGen/Vc ==
  Ua : Inport
  Ub : Inport  Port=2
  Add1 : Sum  Inputs=+-
  Add2 : Sum  Inputs=--
  Add3 : Sum
  Add4 : Sum  Inputs=-+
  Constant : Constant  Value=0.5  OutDataTypeStr=Inherit: Inherit via back propagation
  Product : Product
  Product1 : Product
  sqrt(3)/2 : Constant  Value=0.8660254  OutDataTypeStr=Inherit: Inherit via back propagation
  Va* : Outport
  Vb : Outport  Port=2
  Vb* : Outport  Port=3
  Vc : Outport  Port=4
  Vc* : Outport  Port=5
  wires:
  Add4/1 -> Vc*/1
  Add3/1 -> Vb*/1
  Constant/1 -> Product1/1
  Add1/1 -> Vb/1
  Ub/1 -> Product1/2, Va*/1
  sqrt(3)/2/1 -> Product/2
  Add2/1 -> Vc/1
  Ua/1 -> Product/1
  Product/1 -> Add4/1, Add2/1, Add3/1, Add1/1
  Product1/1 -> Add4/2, Add2/2, Add3/2, Add1/2

== system c28069pmsmfoc_cla/FOC Algorithm/Torque Control Algorithm/Generating Space Vectors/Generating Raw Space Vectors/SVGen/scale ==
  In1 : Inport
  Add : Sum  Inputs=+-
  Constant2 : Constant  Value=0.5  OutDataTypeStr=Inherit: Inherit via back propagation
  Constant3 : Constant  Value=2  OutDataTypeStr=Inherit: Inherit via back propagation
  Product : Product
  Out1 : Outport
  wires:
  Product/1 -> Out1/1
  In1/1 -> Add/1
  Constant3/1 -> Product/2
  Add/1 -> Product/1
  Constant2/1 -> Add/2

== system c28069pmsmfoc_cla/FOC Algorithm/Torque Control Algorithm/Generating Space Vectors/Generating Raw Space Vectors/control/PID Controller ==
  In1 : Inport
  In2 : Inport  Port=2
  Product : Product  OutDataTypeStr=Inherit: Same as first input
  Saturation : Saturate  UpperLimit=maxOutput  LowerLimit=minOutput  LinearizeAsGain=off  ZeroCross=off
  Sum1 : Sum  Inputs=+++
  Sum2 : Sum  Inputs=+-
  Sum3 : Sum  Inputs=+-
  UD_REG3 : Subsystem
  UI_REG3 : Subsystem
  Unit Delay2 : UnitDelay  SampleTime=-1  HasFrameUpgradeWarning=on
  Unit Delay3 : UnitDelay  SampleTime=-1  HasFrameUpgradeWarning=on
  Unit Delay4 : UnitDelay  SampleTime=-1  HasFrameUpgradeWarning=on
  prop_gain : Constant  Value=proportionalGain  OutDataTypeStr=Inherit: Inherit via back propagation
  Out1 : Outport
  wires:
  In2/1 -> Sum2/2
  In1/1 -> Sum2/1
  prop_gain/1 -> Product/2
  Unit Delay2/1 -> UD_REG3/2(PrevOut)
  Sum3/1 -> Unit Delay4/1
  Saturation/1 -> Out1/1, Sum3/1
  Sum1/1 -> Sum3/2, Saturation/1
  UI_REG3/1(UI_REG1) -> Sum1/3, Unit Delay3/1
  UD_REG3/1(Out1) -> Sum1/2
  Product/1 -> Unit Delay2/1, UD_REG3/1(up_reg3), UI_REG3/2(up_reg3), Sum1/1
  Sum2/1 -> Product/1
  Unit Delay3/1 -> UI_REG3/1(OLD_UI_REG3)
  Unit Delay4/1 -> UI_REG3/3(saterr_reg3)

== system c28069pmsmfoc_cla/FOC Algorithm/Torque Control Algorithm/Generating Space Vectors/Generating Raw Space Vectors/control/PID Controller1 ==
  In1 : Inport
  In2 : Inport  Port=2
  Product : Product  OutDataTypeStr=Inherit: Same as first input
  Saturation : Saturate  UpperLimit=maxOutput  LowerLimit=minOutput  LinearizeAsGain=off  ZeroCross=off
  Sum1 : Sum  Inputs=+++
  Sum2 : Sum  Inputs=+-
  Sum3 : Sum  Inputs=+-
  UD_REG3 : Subsystem
  UI_REG3 : Subsystem
  Unit Delay2 : UnitDelay  SampleTime=-1  HasFrameUpgradeWarning=on
  Unit Delay3 : UnitDelay  SampleTime=-1  HasFrameUpgradeWarning=on
  Unit Delay4 : UnitDelay  SampleTime=-1  HasFrameUpgradeWarning=on
  prop_gain : Constant  Value=proportionalGain  OutDataTypeStr=Inherit: Inherit via back propagation
  Out1 : Outport
  wires:
  In2/1 -> Sum2/2
  In1/1 -> Sum2/1
  prop_gain/1 -> Product/2
  Unit Delay2/1 -> UD_REG3/2(PrevOut)
  Sum3/1 -> Unit Delay4/1
  Saturation/1 -> Out1/1, Sum3/1
  Sum1/1 -> Sum3/2, Saturation/1
  UI_REG3/1(UI_REG1) -> Sum1/3, Unit Delay3/1
  UD_REG3/1(Out1) -> Sum1/2
  Product/1 -> Unit Delay2/1, UD_REG3/1(up_reg3), UI_REG3/2(up_reg3), Sum1/1
  Sum2/1 -> Product/1
  Unit Delay3/1 -> UI_REG3/1(OLD_UI_REG3)
  Unit Delay4/1 -> UI_REG3/3(saterr_reg3)

== system c28069pmsmfoc_cla/FOC Algorithm/Torque Control Algorithm/Generating Space Vectors/Generating Raw Space Vectors/control/saturation ==
  In1 : Inport
  In2 : Inport  Port=2
  Demux : Demux  Outputs=2
  Mux3 : Mux  Inputs=2
  Switch1 : Switch  Threshold=1
  Unit Delay : UnitDelay  InitialCondition=[0 0]  SampleTime=-1  HasFrameUpgradeWarning=on
  hypot : Math  Operator=hypot  SignedPower=on  SaturateOnIntegerOverflow=on
  Out1 : Outport
  Out2 : Outport  Port=2
  wires:
  In2/1 -> hypot/2, Mux3/2
  Mux3/1 -> Switch1/3
  Switch1/1 -> Unit Delay/1, Demux/1
  Unit Delay/1 -> Switch1/1
  Demux/1 -> Out1/1
  Demux/2 -> Out2/1
  In1/1 -> hypot/1, Mux3/1
  hypot/1 -> Switch1/2

== system c28069pmsmfoc_cla/FOC Algorithm/Torque Control Algorithm/Input Scaling/Speed and direction are not valid Position will be set to the middle of the Hall quadrant/Extract position from Halls reading. No speed extrapolaiton/Hall Value of 1 ==
  Action Port : ActionPort  ActionPortLabel=case [ 1 ]:
  Constant : Constant  Value=3/12  OutDataTypeStr=fixdt(1,32,17)
  position : Outport
  wires:
  Constant/1 -> position/1

== system c28069pmsmfoc_cla/FOC Algorithm/Torque Control Algorithm/Input Scaling/Speed and direction are not valid Position will be set to the middle of the Hall quadrant/Extract position from Halls reading. No speed extrapolaiton/Hall Value of 2 ==
  Action Port : ActionPort  ActionPortLabel=case [ 2 ]:
  Constant : Constant  Value=7/12  OutDataTypeStr=fixdt(1,32,17)
  position : Outport
  wires:
  Constant/1 -> position/1

== system c28069pmsmfoc_cla/FOC Algorithm/Torque Control Algorithm/Input Scaling/Speed and direction are not valid Position will be set to the middle of the Hall quadrant/Extract position from Halls reading. No speed extrapolaiton/Hall Value of 3 ==
  Action Port : ActionPort  ActionPortLabel=case [ 3 ]:
  Constant : Constant  Value=5/12  OutDataTypeStr=fixdt(1,32,17)
  position : Outport
  wires:
  Constant/1 -> position/1

== system c28069pmsmfoc_cla/FOC Algorithm/Torque Control Algorithm/Input Scaling/Speed and direction are not valid Position will be set to the middle of the Hall quadrant/Extract position from Halls reading. No speed extrapolaiton/Hall Value of 4 ==
  Action Port : ActionPort  ActionPortLabel=case [ 4 ]:
  Constant : Constant  Value=11/12  OutDataTypeStr=fixdt(1,32,17)
  position : Outport
  wires:
  Constant/1 -> position/1

== system c28069pmsmfoc_cla/FOC Algorithm/Torque Control Algorithm/Input Scaling/Speed and direction are not valid Position will be set to the middle of the Hall quadrant/Extract position from Halls reading. No speed extrapolaiton/Hall Value of 5 ==
  Action Port : ActionPort  ActionPortLabel=case [ 5 ]:
  Constant : Constant  Value=1/12  OutDataTypeStr=fixdt(1,32,17)
  position : Outport
  wires:
  Constant/1 -> position/1

== system c28069pmsmfoc_cla/FOC Algorithm/Torque Control Algorithm/Input Scaling/Speed and direction are not valid Position will be set to the middle of the Hall quadrant/Extract position from Halls reading. No speed extrapolaiton/Hall Value of 6 ==
  Action Port : ActionPort  ActionPortLabel=case [ 6 ]:
  Constant : Constant  Value=9/12  OutDataTypeStr=fixdt(1,32,17)
  position : Outport
  wires:
  Constant/1 -> position/1

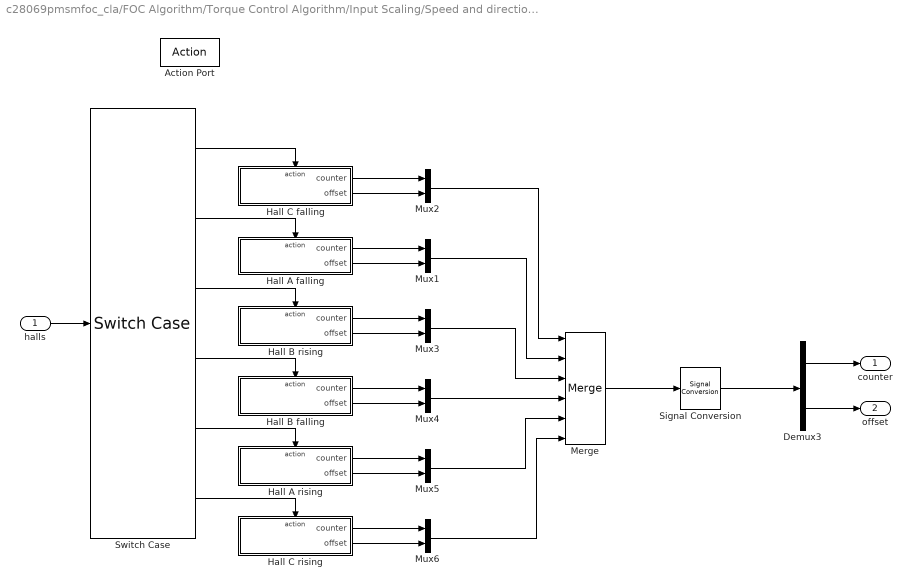
== system c28069pmsmfoc_cla/FOC Algorithm/Torque Control Algorithm/Input Scaling/Speed and direction are valid Use speed to extrapolate position/Extract Position from Halls/Direction 0 Provides offset and counter values ==
  halls : Inport
  Action Port : ActionPort  ActionPortLabel=else
  Demux3 : Demux  Outputs=2
  Hall A falling : Subsystem  TreatAsAtomicUnit=on
  Hall A rising : Subsystem  TreatAsAtomicUnit=on
  Hall B falling : Subsystem  TreatAsAtomicUnit=on
  Hall B rising : Subsystem  TreatAsAtomicUnit=on
  Hall C falling : Subsystem  TreatAsAtomicUnit=on
  Hall C rising : Subsystem  TreatAsAtomicUnit=on
  Merge : Merge  Inputs=6
  Mux{1..6} (6 alike) : Mux  Inputs=2
  Signal Conversion : SignalConversion  OverrideOpt=on
  Switch Case : SwitchCase  CaseConditions={1,2,3,4,5,6}  ShowDefaultCase=off
  counter : Outport
  offset : Outport  Port=2
  wires:
  halls/1 -> Switch Case/1
  Switch Case/2 -> Hall A falling/Action
  Switch Case/5 -> Hall A rising/Action
  Switch Case/6 -> Hall C rising/Action
  Switch Case/1 -> Hall C falling/Action
  Switch Case/3 -> Hall B rising/Action
  Switch Case/4 -> Hall B falling/Action
  Hall C falling/1(counter) -> Mux2/1
  Hall C falling/2(offset) -> Mux2/2
  Hall A falling/1(counter) -> Mux1/1
  Hall A falling/2(offset) -> Mux1/2
  Hall B rising/1(counter) -> Mux3/1
  Hall B rising/2(offset) -> Mux3/2
  Hall B falling/1(counter) -> Mux4/1
  Hall B falling/2(offset) -> Mux4/2
  Hall A rising/1(counter) -> Mux5/1
  Hall A rising/2(offset) -> Mux5/2
  Hall C rising/1(counter) -> Mux6/1
  Hall C rising/2(offset) -> Mux6/2
  Mux2/1 -> Merge/1
  Mux1/1 -> Merge/2
  Mux3/1 -> Merge/3
  Mux4/1 -> Merge/4
  Mux5/1 -> Merge/5
  Mux6/1 -> Merge/6
  Merge/1 -> Signal Conversion/1
  Demux3/2 -> offset/1
  Demux3/1 -> counter/1
  Signal Conversion/1 -> Demux3/1
